simulink model "SimEstanque"  (R2014a)
settings: Solver=ode45  SolverMode=SingleTasking  StartTime=0.0  StopTime=500  RelTol=1e-3
settings Model: CovMetricSettings=dwe  CovHtmlReporting=off  covSaveCumulativeToWorkspaceVar=off  CovSaveSingleToWorkspaceVar=off  CovExternalEMLEnable=on  CovSFcnEnable=on  Creator=rober  LastModifiedBy=rober
settings SolverCC: ZeroCrossAlgorithm=Adaptive
settings DataIOCC: LimitDataPoints=off  SaveFormat=StructureWithTime
settings DebuggingCC: MergeDetectMultiDrivingBlocksExec=error  IgnoredZcDiagnostic=none  SolverPrmCheckMsg=none  FrameProcessingCompatibilityMsg=error  SFUnexpectedBacktrackingDiag=error  SFNoUnconditionalDefaultTransitionDiag=error
settings HardwareCC: ProdBitPerPointer=64  ProdLargestAtomicFloat=Float  ProdIntDivRoundTo=Zero  ProdEndianess=LittleEndian  ProdHWDeviceType=Specified
settings ModelReferenceCC: PropagateSignalLabelsOutOfModel=on
settings SFSimCC: SimUseLocalCustomCode=on
settings RTWCC: RTWUseLocalCustomCode=on
settings GRTTargetCC: TargetLangStandard=C99 (ISO)  GeneratePreprocessorConditionals=Use local settings

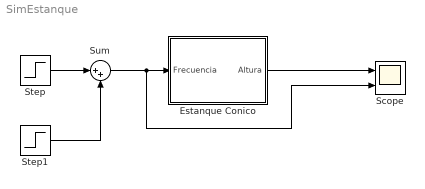
== system SimEstanque ==
  Estanque Conico : Subsystem
  Scope : Scope  NumInputPorts=2
      settings: TimeRange=auto  MaxDataPoints=5000  SaveToWorkspace=off  SaveName=ScopeData  YMin=-12.5~-5  YMax=112.5~5  SampleTime=-1
  Step : Step  Time=25  After=100  SampleTime=0
  Step1 : Step  Time=75  After=-100  SampleTime=0
  Sum : Sum  Inputs=|++
  wires:
  Step/1 -> Sum/1
  Step1/1 -> Sum/2
  Sum/1 -> Scope/2, Estanque Conico/1(Frecuencia)
  Estanque Conico/1(Altura) -> Scope/1

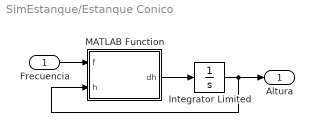
== system SimEstanque/Estanque Conico ==
  Frecuencia : Inport
  Integrator Limited : Integrator  InitialCondition=20  LimitOutput=on  LowerSaturationLimit=0
  MATLAB Function : MATLAB Function  TreatAsAtomicUnit=on
      settings: PermitHierarchicalResolution=ParametersOnly
  Altura : Outport
  wires:
  Integrator Limited/1 -> MATLAB Function/2(h), Altura/1
  MATLAB Function/1(dh) -> Integrator Limited/1
  Frecuencia/1 -> MATLAB Function/1(f)

== matlab function SimEstanque/Estanque Conico/MATLAB Function ==
  data: f input; dh output; h input
function dh = fcn(f,h)
Fin=5.43*f+78.23;
Fout=20.21*sqrt(h);
Num=Fin-Fout;
Den=0.63*h^2+11.4*h+17.1;
dh = real(Num/Den);
